simulink model "IPILCO_SimpleImp_relativeRPY_S"  (R2015b)
settings: Solver=ode45  StartTime=0.0  StopTime=T  RelTol=1e-3
undefined symbols (not defined in the file): accel, addNoise, computeDamping, dt, dt_pilco, dyno, gravload, Hd0, initTrial, jacob0, jacobn, Kd_env, Kp_env, mu0, n, perturbedRobotNF, plant, policy, robot, stateLength, xc, xhole
libraries: roblocks x11
settings Model: Creator=LocalAdmin  LastModifiedBy=vvanspaandonk
settings DataIOCC: SaveFormat=Array
settings DebuggingCC: SolverPrmCheckMsg=warning
settings HardwareCC: ProdBitPerPointer=32  ProdLargestAtomicFloat=None  ProdIntDivRoundTo=Undefined  ProdEndianess=Unspecified  ProdWordSize=32  ProdHWDeviceType=32-bit Generic
settings GRTTargetCC: GeneratePreprocessorConditionals=Disable all
settings ConfigComp: CovModelRefEnable=Off  CovSFcnEnable=off

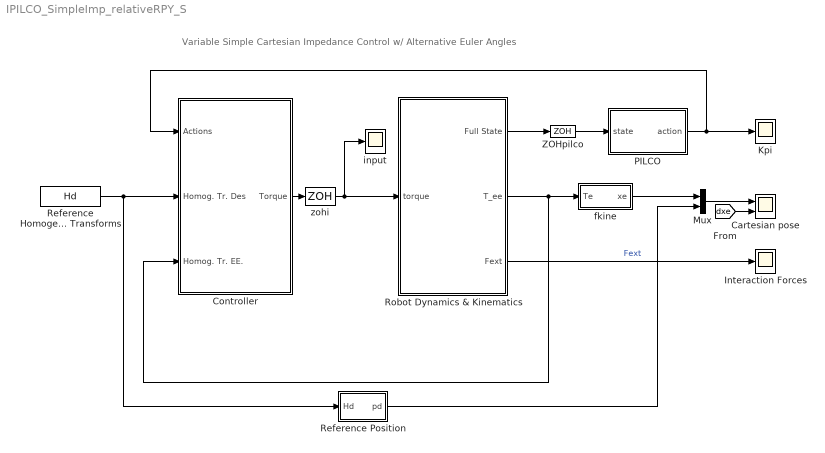
== system IPILCO_SimpleImp_relativeRPY_S ==
  note: Variable Simple Cartesian Impedance Control w/ Alternative Euler Angles
  Cartesian pose : Scope  NumInputPorts=2
  Controller : Subsystem
  Interaction Forces : Scope
  Kpi : Scope
  Mux : Mux  Inputs=2
  PILCO : Subsystem
  Reference Homogenous Transforms : FromWorkspace  VariableName=Hd  SampleTime=dt
  Reference Position : Subsystem
  Robot Dynamics & Kinematics : Subsystem
  ZOHpilco : ZeroOrderHold  SampleTime=dt
  fkine : Subsystem
  input : Scope
  zohi : ZeroOrderHold  SampleTime=dt
  wires:
  Robot Dynamics & Kinematics/3(Fext) -> Interaction Forces/1  "Fext"
  Robot Dynamics & Kinematics/1(Full State) -> ZOHpilco/1
  Controller/1(Torque) -> zohi/1
  Reference Homogenous Transforms/1 -> Reference Position/1(Hd), Controller/2(Homog. Tr. Des)
  Robot Dynamics & Kinematics/2(T_ee) -> Controller/3(Homog. Tr. EE.), fkine/1(Te)
  Reference Position/1(pd) -> Mux/2
  Mux/1 -> Cartesian pose/1
  PILCO/1(action) -> Controller/1(Actions), Kpi/1
  fkine/1(xe) -> Mux/1
  [dxe] -> Cartesian pose/2
  ZOHpilco/1 -> PILCO/1(state)
  zohi/1 -> Robot Dynamics & Kinematics/1(torque), input/1

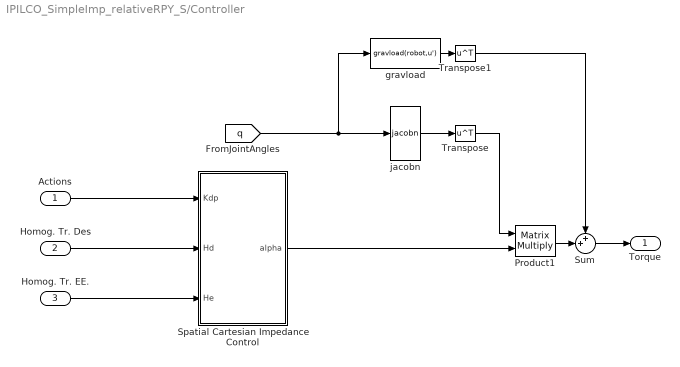
== system IPILCO_SimpleImp_relativeRPY_S/Controller ==
  Actions : Inport
  Homog. Tr. Des : Inport  Port=2
  Homog. Tr. EE. : Inport  Port=3
  Product1 : Product  Multiplication=Matrix(*)
  Spatial Cartesian Impedance Control : Subsystem
  Sum : Sum  Inputs=++|
  Transpose : Math  Operator=transpose  SaturateOnIntegerOverflow=on
  Transpose1 : Math  Operator=transpose  SaturateOnIntegerOverflow=on
  gravload : MATLABFcn  MATLABFcn=gravload(robot,u')  Output1D=off
  jacobn : roblocks/Kinematics/jacobn  robot=robot
  Torque : Outport
  wires:
  Product1/1 -> Sum/2
  Spatial Cartesian Impedance Control/1(alpha) -> Product1/2
  Homog. Tr. EE./1 -> Spatial Cartesian Impedance Control/3(He)
  Actions/1 -> Spatial Cartesian Impedance Control/1(Kdp)
  Homog. Tr. Des/1 -> Spatial Cartesian Impedance Control/2(Hd)
  [q] -> gravload/1, jacobn/1
  jacobn/1 -> Transpose/1
  Transpose/1 -> Product1/1
  gravload/1 -> Transpose1/1
  Transpose1/1 -> Sum/1
  Sum/1 -> Torque/1

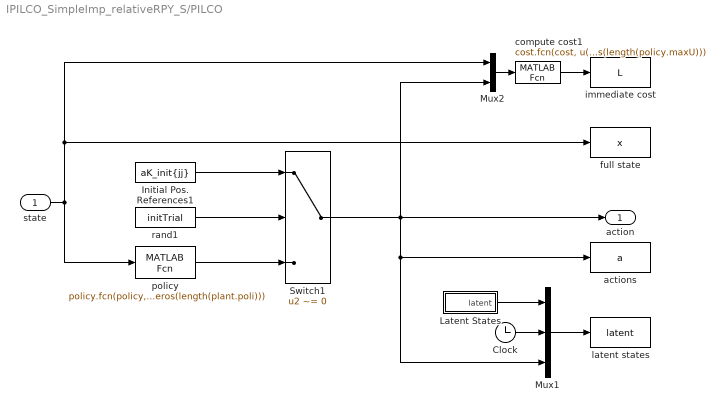
== system IPILCO_SimpleImp_relativeRPY_S/PILCO ==
  state : Inport
  Clock : Clock
  Initial Pos. References1 : FromWorkspace  VariableName=aK_init{jj}  SampleTime=dt_pilco  OutputAfterFinalValue=Holding final value
  Latent States : Subsystem
  Mux1 : Mux  Inputs=3
  Mux2 : Mux  Inputs=2
  Switch1 : Switch  Criteria=u2 ~= 0
  actions : ToWorkspace  VariableName=a  SampleTime=dt_pilco
  compute cost1 : MATLABFcn  MATLABFcn=cost.fcn(cost, u(plant.dyno), zeros(length(plant.dyno)), u(end-length(policy.maxU)+1:end), zeros(length(policy.maxU)))  OutputDimensions=1  Output1D=off
  full state : ToWorkspace  VariableName=x  SampleTime=dt_pilco
  immediate cost : ToWorkspace  VariableName=L  SampleTime=dt_pilco
  latent states : ToWorkspace  VariableName=latent  SampleTime=dt_pilco
  policy : MATLABFcn  MATLABFcn=policy.fcn(policy, u(dyno(plant.poli)), zeros(length(plant.poli)))
  rand1 : Constant  Value=initTrial  SampleTime=dt_pilco
  action : Outport
  wires:
  Mux1/1 -> latent states/1
  compute cost1/1 -> immediate cost/1
  state/1 -> policy/1, Mux2/1, full state/1
  Mux2/1 -> compute cost1/1
  Latent States/1(latent) -> Mux1/1
  rand1/1 -> Switch1/2
  Initial Pos. References1/1 -> Switch1/1
  Switch1/1 -> Mux2/2, action/1, Mux1/3, actions/1
  Clock/1 -> Mux1/2
  policy/1 -> Switch1/3

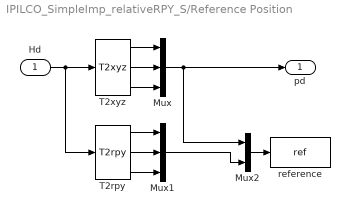
== system IPILCO_SimpleImp_relativeRPY_S/Reference Position ==
  Hd : Inport
  Mux : Mux  Inputs=3
  Mux1 : Mux  Inputs=3
  Mux2 : Mux  Inputs=2
  T2rpy : roblocks/Transform Conversion/T2rpy
  T2xyz : roblocks/Transform Conversion/T2xyz
  reference : ToWorkspace  VariableName=ref  SampleTime=dt_pilco
  pd : Outport
  wires:
  Hd/1 -> T2rpy/1, T2xyz/1
  T2xyz/1 -> Mux/1
  T2xyz/2 -> Mux/2
  T2xyz/3 -> Mux/3
  Mux/1 -> Mux2/1, pd/1
  T2rpy/1 -> Mux1/1
  T2rpy/2 -> Mux1/2
  T2rpy/3 -> Mux1/3
  Mux2/1 -> reference/1
  Mux1/1 -> Mux2/2

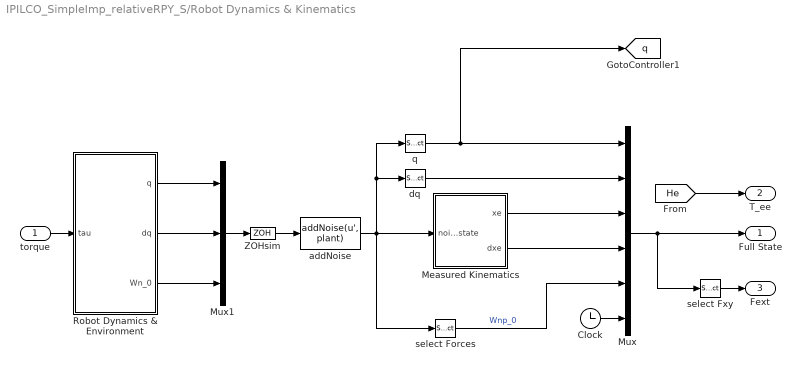
== system IPILCO_SimpleImp_relativeRPY_S/Robot Dynamics & Kinematics ==
  torque : Inport
  Clock : Clock
  Measured Kinematics : Subsystem
  Mux : Mux  Inputs=6
  Mux1 : Mux  Inputs=3
  Robot Dynamics & Environment : Subsystem
  ZOHsim : ZeroOrderHold  SampleTime=dt
  addNoise : MATLABFcn  MATLABFcn=addNoise(u', plant)
  dq : Selector  InputPortWidth=2*robot.n+6  IndexOptions=Index vector (dialog)  Indices=[robot.n+1:2*robot.n]  OutputSizes=1
  q : Selector  InputPortWidth=2*robot.n+6  IndexOptions=Index vector (dialog)  Indices=[1:robot.n]  OutputSizes=1
  select Forces : Selector  InputPortWidth=2*robot.n+6  IndexOptions=Index vector (dialog)  Indices=[2*robot.n+1:2*robot.n+6]  OutputSizes=1
  select Fxy : Selector  InputPortWidth=stateLength  IndexOptions=Index vector (dialog)  Indices=[stateLength-6:1:stateLength-1]  OutputSizes=1
  Full State : Outport
  T_ee : Outport  Port=2
  Fext : Outport  Port=3
  tag scope: q=global
  wires:
  torque/1 -> Robot Dynamics & Environment/1(tau)
  Measured Kinematics/1(xe) -> Mux/3
  Measured Kinematics/2(dxe) -> Mux/4
  select Fxy/1 -> Fext/1
  q/1 -> [q], Mux/1
  dq/1 -> Mux/2
  Robot Dynamics & Environment/1(q) -> Mux1/1
  Robot Dynamics & Environment/2(dq) -> Mux1/2
  Mux1/1 -> ZOHsim/1
  Robot Dynamics & Environment/3(Wn_0) -> Mux1/3
  Mux/1 -> Full State/1, select Fxy/1
  select Forces/1 -> Mux/5  "Wnp_0"
  [He] -> T_ee/1
  ZOHsim/1 -> addNoise/1
  addNoise/1 -> q/1, dq/1, select Forces/1, Measured Kinematics/1(noisy state)
  Clock/1 -> Mux/6

== system IPILCO_SimpleImp_relativeRPY_S/fkine ==
  Te : Inport
  Mux1 : Mux  Inputs=6
  T2rpy : roblocks/Transform Conversion/T2rpy
  T2xyz : roblocks/Transform Conversion/T2xyz
  xe : Outport
  wires:
  Te/1 -> T2xyz/1, T2rpy/1
  T2xyz/2 -> Mux1/2
  T2rpy/1 -> Mux1/4
  T2xyz/1 -> Mux1/1
  T2rpy/2 -> Mux1/5
  Mux1/1 -> xe/1
  T2xyz/3 -> Mux1/3
  T2rpy/3 -> Mux1/6

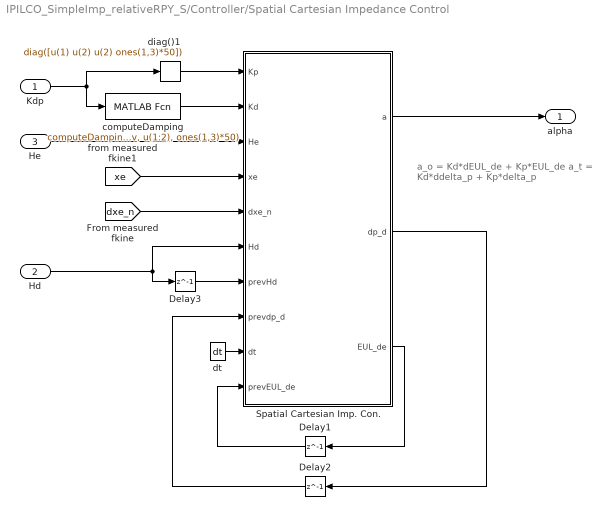
== system IPILCO_SimpleImp_relativeRPY_S/Controller/Spatial Cartesian Impedance Control ==
  note: a_o = Kd*dEUL_de + Kp*EUL_de
      |
      | a_t = Kd*ddelta_p + Kp*delta_p
  Kdp : Inport
  Hd : Inport  Port=2
  He : Inport  Port=3
  Delay1 : Delay  DelayLength=1  InitialCondition=0  SampleTime=dt
  Delay2 : Delay  DelayLength=1  InitialCondition=0  SampleTime=dt
  Delay3 : Delay  DelayLength=1  InitialCondition=Hd0  SampleTime=dt
  Spatial Cartesian Imp. Con. : MATLAB Function  TreatAsAtomicUnit=on
  computeDamping : MATLABFcn  MATLABFcn=computeDamping(Kp_env, u(1:2), ones(1,3)*50)  OutputDimensions=[6 6]  Output1D=off
  diag()1 : MATLABFcn  MATLABFcn=diag([u(1) u(2) u(2) ones(1,3)*50])  OutputDimensions=[6 6]  Output1D=off
  dt : Constant  Value=dt  SampleTime=dt
  alpha : Outport
  wires:
  dt/1 -> Spatial Cartesian Imp. Con./9(dt)
  Hd/1 -> Spatial Cartesian Imp. Con./6(Hd), Delay3/1
  He/1 -> Spatial Cartesian Imp. Con./3(He)
  diag()1/1 -> Spatial Cartesian Imp. Con./1(Kp)
  Spatial Cartesian Imp. Con./2(dp_d) -> Delay2/1
  Delay2/1 -> Spatial Cartesian Imp. Con./8(prevdp_d)
  Delay3/1 -> Spatial Cartesian Imp. Con./7(prevHd)
  [dxe_n] -> Spatial Cartesian Imp. Con./5(dxe_n)
  [xe] -> Spatial Cartesian Imp. Con./4(xe)
  Spatial Cartesian Imp. Con./1(a) -> alpha/1
  computeDamping/1 -> Spatial Cartesian Imp. Con./2(Kd)
  Kdp/1 -> diag()1/1, computeDamping/1
  Spatial Cartesian Imp. Con./3(EUL_de) -> Delay1/1
  Delay1/1 -> Spatial Cartesian Imp. Con./10(prevEUL_de)

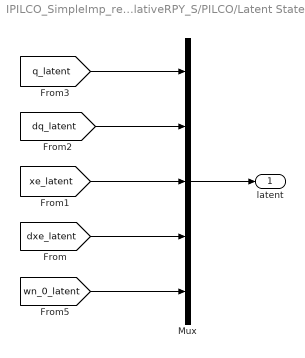
== system IPILCO_SimpleImp_relativeRPY_S/PILCO/Latent States ==
  Mux : Mux  Inputs=5
  latent : Outport
  wires:
  [dq_latent] -> Mux/2
  [q_latent] -> Mux/1
  [wn_0_latent] -> Mux/5
  [dxe_latent] -> Mux/4
  [xe_latent] -> Mux/3
  Mux/1 -> latent/1

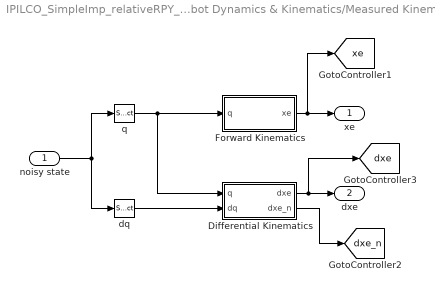
== system IPILCO_SimpleImp_relativeRPY_S/Robot Dynamics & Kinematics/Measured Kinematics ==
  noisy state : Inport
  Differential Kinematics : Subsystem
  Forward Kinematics : Subsystem
  dq : Selector  InputPortWidth=2*robot.n + 6  IndexOptions=Index vector (dialog)  Indices=[robot.n+1:2*robot.n]  OutputSizes=1
  q : Selector  InputPortWidth=2*robot.n+6  IndexOptions=Index vector (dialog)  Indices=[1:robot.n]  OutputSizes=1
  xe : Outport
  dxe : Outport  Port=2
  tag scope: dxe=global, dxe_n=global, xe=global
  wires:
  q/1 -> Differential Kinematics/1(q), Forward Kinematics/1(q)
  noisy state/1 -> q/1, dq/1
  dq/1 -> Differential Kinematics/2(dq)
  Forward Kinematics/1(xe) -> [xe], xe/1
  Differential Kinematics/2(dxe_n) -> [dxe_n]
  Differential Kinematics/1(dxe) -> [dxe], dxe/1

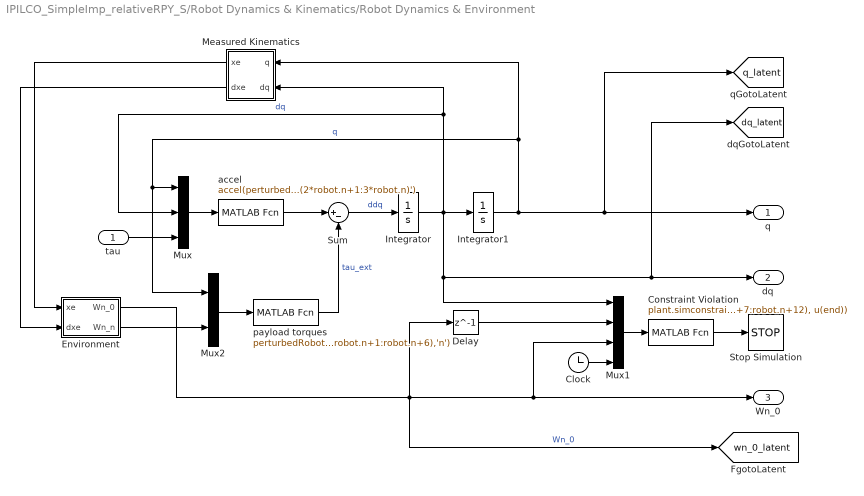
== system IPILCO_SimpleImp_relativeRPY_S/Robot Dynamics & Kinematics/Robot Dynamics & Environment ==
  tau : Inport
  Clock : Clock
  Constraint Violation : MATLABFcn  MATLABFcn=plant.simconstraint(u(1:robot.n), u(robot.n+1:robot.n+6), u(robot.n+7:robot.n+12), u(end))
  Delay : Delay  DelayLength=1  InitialCondition=0  SampleTime=dt
  Environment : Subsystem
  Integrator : Integrator
  Integrator1 : Integrator  InitialCondition=mu0(1:robot.n)
  Measured Kinematics : Subsystem
  Mux : Mux  Inputs=3
  Mux1 : Mux
  Mux2 : Mux  Inputs=2
  Stop Simulation : Stop
  Sum : Sum  Inputs=|+-
  accel : MATLABFcn  MATLABFcn=accel(perturbedRobotNF,u(1:robot.n)',u(robot.n+1:2*robot.n)',u(2*robot.n+1:3*robot.n)')
  payload torques : MATLABFcn  MATLABFcn=perturbedRobotNF.pay(u(1:robot.n)',u(robot.n+1:robot.n+6),'n')
  q : Outport
  dq : Outport  Port=2
  Wn_0 : Outport  Port=3
  tag scope: dq_latent=global, q_latent=global, wn_0_latent=global
  wires:
  accel/1 -> Sum/1
  Mux/1 -> accel/1
  tau/1 -> Mux/3
  payload torques/1 -> Sum/2  "tau_ext"
  Sum/1 -> Integrator/1  "ddq"
  Mux1/1 -> Constraint Violation/1
  Constraint Violation/1 -> Stop Simulation/1
  Measured Kinematics/2(dxe) -> Environment/2(dxe)
  Integrator/1 -> Mux/2, Measured Kinematics/2(dq), Integrator1/1, Mux1/1, [dq_latent], dq/1  "dq"
  Integrator1/1 -> Measured Kinematics/1(q), Mux2/1, Mux/1, [q_latent], q/1  "q"
  Environment/1(Wn_0) -> Delay/1, [wn_0_latent], Mux1/3, Wn_0/1  "Wn_0"
  Mux2/1 -> payload torques/1
  Environment/2(Wn_n) -> Mux2/2
  Measured Kinematics/1(xe) -> Environment/1(xe)
  Delay/1 -> Mux1/2
  Clock/1 -> Mux1/4

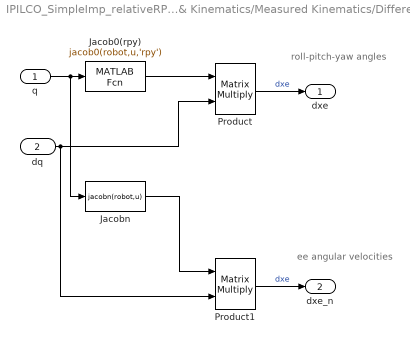
== system IPILCO_SimpleImp_relativeRPY_S/Robot Dynamics & Kinematics/Measured Kinematics/Differential Kinematics ==
  note: roll-pitch-yaw
      | angles
  note: ee angular
      | velocities
  q : Inport
  dq : Inport  Port=2
  Jacob0(rpy) : MATLABFcn  MATLABFcn=jacob0(robot,u,'rpy')  OutputDimensions=[6 n]  Output1D=off
  Jacobn : MATLABFcn  MATLABFcn=jacobn(robot,u)  OutputDimensions=[6 n]  Output1D=off
  Product : Product  Multiplication=Matrix(*)
  Product1 : Product  Multiplication=Matrix(*)
  dxe : Outport
  dxe_n : Outport  Port=2
  wires:
  q/1 -> Jacobn/1, Jacob0(rpy)/1
  Product/1 -> dxe/1  "dxe"
  Jacob0(rpy)/1 -> Product/1
  Jacobn/1 -> Product1/1
  Product1/1 -> dxe_n/1  "dxe"
  dq/1 -> Product1/2, Product/2

== system IPILCO_SimpleImp_relativeRPY_S/Robot Dynamics & Kinematics/Measured Kinematics/Forward Kinematics ==
  q : Inport
  Mux : Mux  Inputs=6
  T2rpy : roblocks/Transform Conversion/T2rpy
  T2xyz : roblocks/Transform Conversion/T2xyz
  fkine : roblocks/Kinematics/fkine  robot=robot
  xe : Outport
  tag scope: He=global
  wires:
  T2xyz/3 -> Mux/3
  T2rpy/3 -> Mux/6
  T2rpy/1 -> Mux/4
  T2xyz/2 -> Mux/2
  q/1 -> fkine/1
  fkine/1 -> T2rpy/1, T2xyz/1, [He]
  T2xyz/1 -> Mux/1
  T2rpy/2 -> Mux/5
  Mux/1 -> xe/1

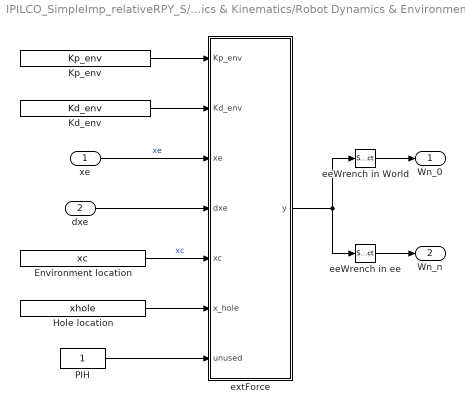
== system IPILCO_SimpleImp_relativeRPY_S/Robot Dynamics & Kinematics/Robot Dynamics & Environment/Environment ==
  xe : Inport
  dxe : Inport  Port=2
  Environment location : Constant  Value=xc  SampleTime=dt
  Hole location : Constant  Value=xhole  SampleTime=dt
  Kd_env : Constant  Value=Kd_env
  Kp_env : Constant  Value=Kp_env
  PIH : Constant  SampleTime=dt
  eeWrench in World : Selector  InputPortWidth=12  IndexOptions=Index vector (dialog)  Indices=1:1:6  OutputSizes=1
  eeWrench in ee : Selector  InputPortWidth=12  IndexOptions=Index vector (dialog)  Indices=7:1:12  OutputSizes=1
  extForce : MATLAB Function  TreatAsAtomicUnit=on
  Wn_0 : Outport
  Wn_n : Outport  Port=2
  wires:
  Environment location/1 -> extForce/5(xc)  "xc"
  xe/1 -> extForce/3(xe)  "xe"
  Kp_env/1 -> extForce/1(Kp_env)
  Kd_env/1 -> extForce/2(Kd_env)
  dxe/1 -> extForce/4(dxe)
  extForce/1(y) -> eeWrench in World/1, eeWrench in ee/1
  PIH/1 -> extForce/7(unused)
  eeWrench in World/1 -> Wn_0/1
  eeWrench in ee/1 -> Wn_n/1
  Hole location/1 -> extForce/6(x_hole)

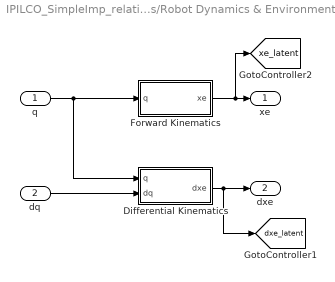
== system IPILCO_SimpleImp_relativeRPY_S/Robot Dynamics & Kinematics/Robot Dynamics & Environment/Measured Kinematics ==
  q : Inport
  dq : Inport  Port=2
  Differential Kinematics : Subsystem
  Forward Kinematics : Subsystem
  xe : Outport
  dxe : Outport  Port=2
  tag scope: dxe_latent=global, xe_latent=global
  wires:
  q/1 -> Differential Kinematics/1(q), Forward Kinematics/1(q)
  dq/1 -> Differential Kinematics/2(dq)
  Differential Kinematics/1(dxe) -> [dxe_latent], dxe/1
  Forward Kinematics/1(xe) -> [xe_latent], xe/1

== system IPILCO_SimpleImp_relativeRPY_S/Robot Dynamics & Kinematics/Robot Dynamics & Environment/Measured Kinematics/Differential Kinematics ==
  q : Inport
  dq : Inport  Port=2
  Jacob0(rpy) : MATLABFcn  MATLABFcn=jacob0(robot,u,'rpy')  OutputDimensions=[6 n]  Output1D=off
  Product : Product  Multiplication=Matrix(*)
  dxe : Outport
  wires:
  q/1 -> Jacob0(rpy)/1
  Product/1 -> dxe/1  "dxe"
  dq/1 -> Product/2
  Jacob0(rpy)/1 -> Product/1

== system IPILCO_SimpleImp_relativeRPY_S/Robot Dynamics & Kinematics/Robot Dynamics & Environment/Measured Kinematics/Forward Kinematics ==
  q : Inport
  Mux : Mux  Inputs=6
  T2rpy : roblocks/Transform Conversion/T2rpy
  T2xyz : roblocks/Transform Conversion/T2xyz
  fkine : roblocks/Kinematics/fkine  robot=robot
  xe : Outport
  wires:
  T2xyz/3 -> Mux/3
  T2rpy/3 -> Mux/6
  T2rpy/1 -> Mux/4
  T2xyz/2 -> Mux/2
  q/1 -> fkine/1
  fkine/1 -> T2rpy/1, T2xyz/1
  T2xyz/1 -> Mux/1
  T2rpy/2 -> Mux/5
  Mux/1 -> xe/1

== matlab function IPILCO_SimpleImp_relativeRPY_S/Controller/Spatial Cartesian Impedance Control/Spatial Cartesian Imp. Con. ==
  data: a output size=[6 1]; dp_d output size=[3 1]; Kp input size=[6 6]; Kd input size=[6 6]; He input size=[4 4]; xe input size=[6 1]; dxe_n input size=[6 1]; Hd input size=[4 4]; prevHd input size=[4 4]; prevdp_d input size=[3 1]; dt input size=1; EUL_de output; prevEUL_de input
function [a, dp_d, EUL_de] = altEulCartImpControl(Kp, Kd, He, xe, dxe_n, Hd, prevHd, prevdp_d, dt, prevEUL_de)
% Computes modified euler angles EUL_de
%
% Outputs
%               - a             computed impedance actions in Cartesian space
%               - Ta            Transformation between analytical and geometric Jacobian
%               - T_e           transformation of Euler angle deriv. to angular vel. of ee-frame
%               - dT_e          time derivative of transf. matrix.
%
% Inputs:
%               - Kp                diagonal stiffness matrix
%               - Kd                diagonal damping matrix
%               - He                current homog. transf. of ee-frame
%               - Hd                desired homog. transf.
%               - xe                current end-effector pose
%               - dxe_n             current end-effector velocity (ee-frame
%               - prevHd            previous desired homog. transf.
%               - prevdp_d          previous desired translational velocity
%               - prevEUL_de        previous relative euler angles
%               - prevHe            previous homog. transf. of ee-frame
%               - dt                sampling time
%
% Code by Victor van Spaandonk
% May 2016
%

%% Prepare inputs
R_e = tr2rt(He);         % Rotation of ee-frame          (referred to base)
R_d = tr2rt(Hd);          % Rotation of desired frame     (referred to base)

%% Translational Actions
p_e = xe(1:3);                  % current ee pos.
p_d = transl(Hd);               % current desired pos.
delta_p = (p_d - p_e);          % positional error

dp_e = dxe_n(1:3);              % current ee transl vel.
prevp_d = transl(prevHd);       % previous desired postion
dp_d = (p_d - prevp_d)./dt;     % current desired velocity
ddelta_p = (dp_d - dp_e);       % velocity error

% ddp_d = (dp_d - prevdp_d)./dt;  % current desired acceleration

a_t = (Kd(1:3,1:3)*ddelta_p + Kp(1:3,1:3)*delta_p);

%% Rotational Actions
% EUL_e = my_tr2rpy(R_e,'xyz');           % Euler angles of ee-frame

Re_d = R_e'*R_d;                        % mutual orientation of ee-frame w.r.t. desired frame
EUL_de = my_tr2rpy(Re_d,'xyz')';        % extract EULER rpy-angles (xyz)
dEUL_de = (EUL_de - prevEUL_de)/dt;

% omega_e = dxe_n(4:6);                   % angular velocity of ee-frame
% omega_d = ((my_tr2rpy(Hd,'xyz') - my_tr2rpy(prevHd,'xyz'))./dt)';
% deltaEuler = omega_d - omega_e;

a_o = (Kd(4:6,4:6)*dEUL_de + Kp(4:6,4:6)*EUL_de);

a = [a_t; a_o];

== matlab function IPILCO_SimpleImp_relativeRPY_S/Robot Dynamics & Kinematics/Robot Dynamics & Environment/Environment/extForce ==
  data: Kp_env input; y output; Kd_env input; xe input; dxe input; xc input; x_hole input; unused input
function y = extForcefcn(Kp_env, Kd_env, xe, dxe, xc, x_hole, ~)
%Simulate external forces when performing PIH insertion.
% Environment is modelled as a spring+directional damping
%
% 1) Fext = Wrench on ee, expressed in perpendicular ee-frame
% 2) transform wrench from pee-frame to ee-frame
% 3) transform back to joints with geometric jacobian in ee-frame
%
%% Inits
persistent INHOLE INSERTED;
if isempty(INHOLE)
    INHOLE = 0;
end
if isempty(INSERTED)
    INSERTED = false;
end
Fext = zeros(6,1);
CONTACT = 0;

%% Constants
cf_v = 0;               % viscous friction coefficient
insertStiffness = 500;  % stiffness to overcome insertion.
r_hole = 0.005;          % tolerance per side of the peg
ywall_l = x_hole(2)+r_hole; ywall_r = x_hole(2)-r_hole;

%% Homogeneous Transformations
R0_n = my_rpy2r(xe(4:6)','xyz');    % roll-pitch-yaw angles of ee-frame w.r.t. base frame
p0_n = xe(1:3);
H0_n = rt2tr(R0_n,p0_n);                            % transform from world to ee-frame (fkine)

% H0_np = rt2tr(eye(3), xe(1:3));                     % homog. transf. from world-frame to ee-frame perpendicular to wall
% Hnp_0 = rt2tr(eye(3), -xe(1:3));
% Hnp_n = H0_n*Hnp_0;

%% determine state
% R0_np = eye(3);
% rpy = tr2diff(R0_np,R0_n);          % roll-pitch-yaw angles between base-frame and ee-frame
% rpy = xe(4:6);

if xe(1) > xc(1)
    CONTACT = 1;
    if xe(2) > ywall_r && xe(2) < ywall_l %&& ((rpy(2)+rpy(3)) < 2*pi*(10/360))  % pitch+yaw should be less than 5 degrees
        INHOLE = 1;
    end
    if xe(1) > x_hole(1) + 0.033    % past insertion resistance
        INSERTED = true;
    end
end

if xe(2) > xc(2)        % contact with surrounding box
    Fext(2) = Kp_env(2)*(xe(2)-xc(2));
elseif xe(2) < -xc(2)
    Fext(2) = Kp_env(2)*(-xe(2)-xc(2));
end

%% Insertion Forces
if CONTACT && ~INHOLE            % wall contact
    
    Fext(1) = Kp_env(1)*(xe(1)-xc(1));              % stiffness force -X
    if dxe(1) > 0
        Fext(1) = Fext(1) + Kd_env(1)*dxe(1);       % damping force   -X
    end
    
    %     Fn = cf_v * Fext(1);                    % normal force
    %     Fext(2) = Fext(2) + Fn*sign(dxe(2));   % Coulomb friction +-Y
    %     Fext(3) = Fext(3) + Fn*sign(dxe(3));   % Couloumb friction +-Z
    
    Fext(2) = Fext(2) + cf_v*dxe(2);   % viscous friction +-Y
    Fext(3) = Fext(3) + cf_v*dxe(3);   % viscous friction +-Z
    
elseif CONTACT && INHOLE    % peg is in hole
    
    % end of hole
    if xe(1) > x_hole(1) + 0.05;
        Fext(1) = Fext(1) + Kp_env(1)*(xe(1)-(x_hole(1) + 0.05)); % stiffness force -X
        if dxe(1) > 0
            Fext(1) = Fext(1) + Kd_env(1)*dxe(1);       % damping force   -X
        end
    end
    
    if xe(1) > x_hole(1)+0.016 && xe(1) < x_hole(1)+0.033 && ~INSERTED
        Fext(1) = Fext(1) + insertStiffness*(xe(1) - (x_hole(1)+0.016));   % insertion resistance -X
    end
    
    % Simulate walls:
    if xe(2) > ywall_l          %&& xe(1) < x_hole(1)+0.033
        Fext(2) = Fext(2) + Kp_env(2)*(xe(2)-ywall_l);            % perp. wall stiffness -Y
        if dxe(2) > 0
            Fext(2) = Fext(2) + Kd_env(2)*dxe(2);       % damping force   -Y
        end
        
        Fext(1) = Fext(1) + Fext(2)*cf_v*dxe(1);                  % friction force -X
        
    elseif xe(2) < ywall_r      % && xe(1) < x_hole(1)+0.033
        Fext(2) = Fext(2) + Kp_env(2)*(xe(2)-ywall_r);  % perp. wall stiffness -Y
        if dxe(2) < 0
            Fext(2) = Fext(2) + Kd_env(2)*dxe(2);       % damping force   -Y
        end
        
        Fext(1) = Fext(1) + Fext(2)*cf_v*dxe(1);        % wall friction force -X
    end
end

W0_n = -Fext;                     % wrench in world frame
Wn_n = wtrans(H0_n, W0_n);       % wrench in ee-frame
y = [W0_n; Wn_n];
